simulink model "linmodel_eq1_val"  (R2019a)
settings: Solver=VariableStepAuto  StartTime=0.0  StopTime=30  RelTol=1e-3
undefined symbols (not defined in the file): A_eq1, B, C, Continuous, T, Time
libraries: ctrlSharedLib x1
settings Model: Creator=jessi  LastModifiedBy=jessi

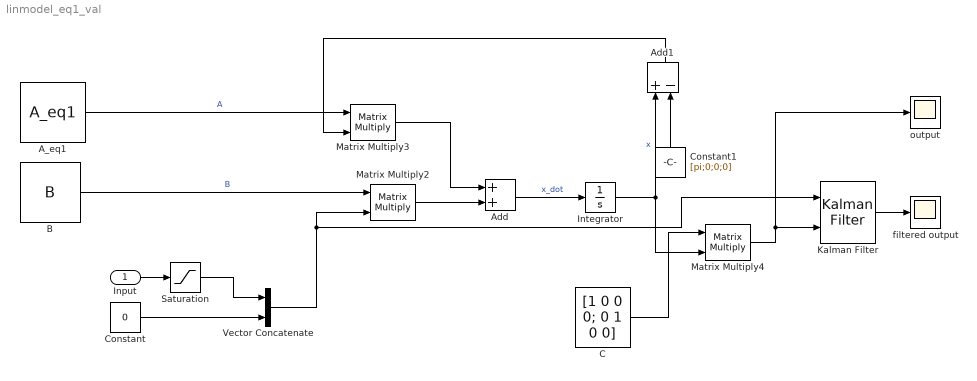
== system linmodel_eq1_val ==
  Input : Inport
  A_eq1 : Constant  Value=A_eq1
  Add : Sum
  Add1 : Sum  Inputs=+-
  B : Constant  Value=B
  C : Constant  Value=|
      | [1 0 0 0;
      | 0 1 0 0]
  Constant : Constant  Value=0
  Constant1 : Constant  Value=[pi;0;0;0]  SampleTime=-1
  Integrator : Integrator  InitialCondition=[pi;0;0;0]
  Kalman Filter : ctrlSharedLib/Kalman Filter  TimeDomain=Continuous-Time  UseCurrentEstimator=on  ModelSource=Individual A, B, C, D matrices  ModelSourceVariable=ss(0.95,1,1,0,1)  A=A_eq1  B=B  C=C  D=0  NumberOfStates=1  NumberOfInputs=1  NumberOfOutputs=1  InitialEstimateSource=Dialog  X0=[pi;0;0;0]  P0=10  UseK=off  UseGH=off  NumberOfProcessNoiseInputs=1  G=1  TimeInvariantG=on  H=0  TimeInvariantH=on  Q=diag([1, 1, 10, 10])  TimeInvariantQ=on  R=diag([0.1, 0.1])  TimeInvariantR=on  N=0  TimeInvariantN=on  AddInputPort=on  AddEnablePort=off  OutputEstimatedY=off  OutputP=off  Ts=T
      settings: SourceProductBaseCode=CT
  Matrix Multiply2 : Product  Multiplication=Matrix(*)
  Matrix Multiply3 : Product  Multiplication=Matrix(*)
  Matrix Multiply4 : Product  Multiplication=Matrix(*)
  Saturation : Saturate  UpperLimit=1  LowerLimit=-1
  Vector Concatenate : Concatenate
  filtered output : Scope
  output : Scope
  wires:
  B/1 -> Matrix Multiply2/1  "B"
  Matrix Multiply2/1 -> Add/2
  A_eq1/1 -> Matrix Multiply3/1  "A"
  Add/1 -> Integrator/1  "x_dot"
  Integrator/1 -> Matrix Multiply4/2, Add1/1  "x"
  Matrix Multiply3/1 -> Add/1
  Matrix Multiply4/1 -> Kalman Filter/2, output/1
  Input/1 -> Saturation/1
  Constant/1 -> Vector Concatenate/2
  C/1 -> Matrix Multiply4/1
  Saturation/1 -> Vector Concatenate/1
  Kalman Filter/1 -> filtered output/1
  Constant1/1 -> Add1/2
  Add1/1 -> Matrix Multiply3/2
  Vector Concatenate/1 -> Matrix Multiply2/2, Kalman Filter/1
